simulink model "stronglyConnectedComponentsTest"  (R2021a)
settings: Solver=VariableStepDiscrete  StartTime=0.0  StopTime=10.0  RelTol=1e-3
settings Model: Creator=cyarp  LastModifiedBy=cyarp

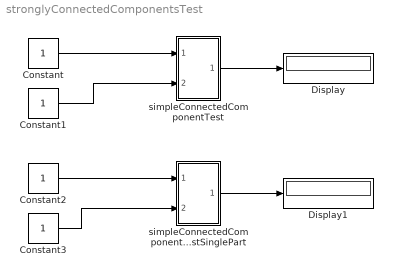
== system stronglyConnectedComponentsTest ==
  Constant{,1..3} (4 alike) : Constant  OutDataTypeStr=single
  Display : Display
  Display1 : Display
  simpleConnectedComponentTest : Subsystem
  simpleConnectedComponentTestSinglePart : Subsystem
  wires:
  Constant/1 -> simpleConnectedComponentTest/1(In1)
  Constant1/1 -> simpleConnectedComponentTest/2(In2)
  simpleConnectedComponentTest/1(Out1) -> Display/1
  Constant2/1 -> simpleConnectedComponentTestSinglePart/1(In1)
  Constant3/1 -> simpleConnectedComponentTestSinglePart/2(In2)
  simpleConnectedComponentTestSinglePart/1(Out1) -> Display1/1

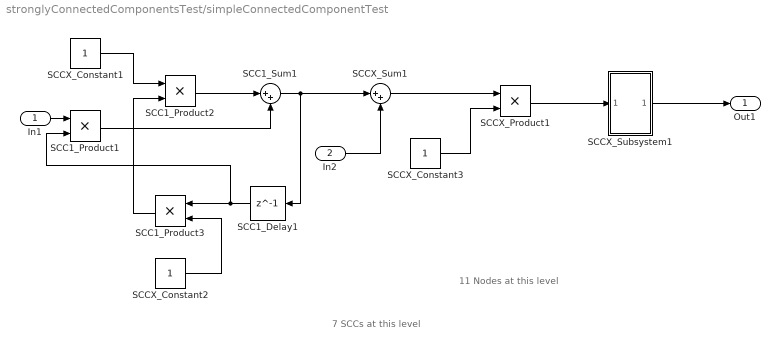
== system stronglyConnectedComponentsTest/simpleConnectedComponentTest ==
  note: 7 SCCs at this level
  note: 11 Nodes at this level
  In1 : Inport
  In2 : Inport  Port=2
  SCC1_Delay1 : Delay  DelayLength=1
  SCC1_Product1 : Product
  SCC1_Product2 : Product
  SCC1_Product3 : Product
  SCC1_Sum1 : Sum  Inputs=|++
  SCCX_Constant1 : Constant  OutDataTypeStr=single
  SCCX_Constant2 : Constant  OutDataTypeStr=single
  SCCX_Constant3 : Constant  OutDataTypeStr=single
  SCCX_Product1 : Product
  SCCX_Subsystem1 : Subsystem
  SCCX_Sum1 : Sum  Inputs=|++
  Out1 : Outport
  wires:
  SCC1_Product1/1 -> SCC1_Sum1/2
  SCC1_Delay1/1 -> SCC1_Product3/1, SCC1_Product1/2
  In2/1 -> SCCX_Sum1/2
  SCCX_Subsystem1/1(Out1) -> Out1/1
  SCC1_Sum1/1 -> SCCX_Sum1/1, SCC1_Delay1/1
  In1/1 -> SCC1_Product1/1
  SCC1_Product2/1 -> SCC1_Sum1/1
  SCCX_Sum1/1 -> SCCX_Product1/1
  SCC1_Product3/1 -> SCC1_Product2/2
  SCCX_Constant1/1 -> SCC1_Product2/1
  SCCX_Constant2/1 -> SCC1_Product3/2
  SCCX_Constant3/1 -> SCCX_Product1/2
  SCCX_Product1/1 -> SCCX_Subsystem1/1(In1)

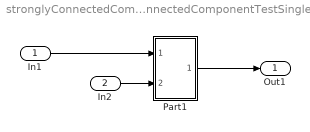
== system stronglyConnectedComponentsTest/simpleConnectedComponentTestSinglePart ==
  In1 : Inport
  In2 : Inport  Port=2
  Part1 : Subsystem
  Out1 : Outport
  wires:
  In1/1 -> Part1/1(In1)
  In2/1 -> Part1/2(In2)
  Part1/1(Out1) -> Out1/1

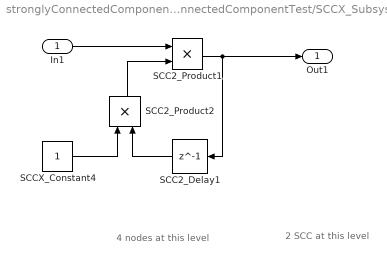
== system stronglyConnectedComponentsTest/simpleConnectedComponentTest/SCCX_Subsystem1 ==
  note: 2 SCC at this level
  note: 4 nodes at this level
  In1 : Inport
  SCC2_Delay1 : Delay  DelayLength=1
  SCC2_Product1 : Product
  SCC2_Product2 : Product
  SCCX_Constant4 : Constant  OutDataTypeStr=single
  Out1 : Outport
  wires:
  SCC2_Delay1/1 -> SCC2_Product2/2
  SCC2_Product1/1 -> Out1/1, SCC2_Delay1/1
  In1/1 -> SCC2_Product1/1
  SCC2_Product2/1 -> SCC2_Product1/2
  SCCX_Constant4/1 -> SCC2_Product2/1

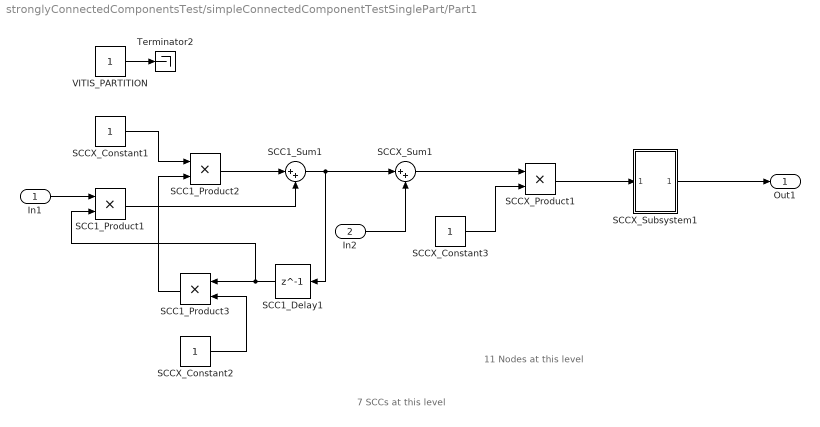
== system stronglyConnectedComponentsTest/simpleConnectedComponentTestSinglePart/Part1 ==
  note: 7 SCCs at this level
  note: 11 Nodes at this level
  In1 : Inport
  In2 : Inport  Port=2
  SCC1_Delay1 : Delay  DelayLength=1
  SCC1_Product1 : Product
  SCC1_Product2 : Product
  SCC1_Product3 : Product
  SCC1_Sum1 : Sum  Inputs=|++
  SCCX_Constant1 : Constant  OutDataTypeStr=single
  SCCX_Constant2 : Constant  OutDataTypeStr=single
  SCCX_Constant3 : Constant  OutDataTypeStr=single
  SCCX_Product1 : Product
  SCCX_Subsystem1 : Subsystem
  SCCX_Sum1 : Sum  Inputs=|++
  Terminator2 : Terminator
  VITIS_PARTITION : Constant
  Out1 : Outport
  wires:
  SCCX_Constant3/1 -> SCCX_Product1/2
  SCCX_Subsystem1/1(Out1) -> Out1/1
  SCC1_Product2/1 -> SCC1_Sum1/1
  SCC1_Delay1/1 -> SCC1_Product3/1, SCC1_Product1/2
  SCC1_Product3/1 -> SCC1_Product2/2
  SCCX_Constant2/1 -> SCC1_Product3/2
  In2/1 -> SCCX_Sum1/2
  SCC1_Sum1/1 -> SCCX_Sum1/1, SCC1_Delay1/1
  SCC1_Product1/1 -> SCC1_Sum1/2
  In1/1 -> SCC1_Product1/1
  SCCX_Constant1/1 -> SCC1_Product2/1
  SCCX_Sum1/1 -> SCCX_Product1/1
  SCCX_Product1/1 -> SCCX_Subsystem1/1(In1)
  VITIS_PARTITION/1 -> Terminator2/1

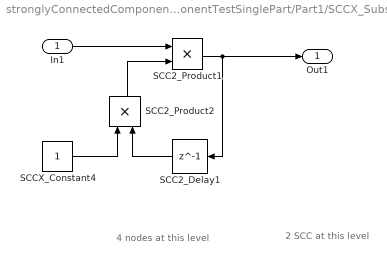
== system stronglyConnectedComponentsTest/simpleConnectedComponentTestSinglePart/Part1/SCCX_Subsystem1 ==
  note: 2 SCC at this level
  note: 4 nodes at this level
  In1 : Inport
  SCC2_Delay1 : Delay  DelayLength=1
  SCC2_Product1 : Product
  SCC2_Product2 : Product
  SCCX_Constant4 : Constant  OutDataTypeStr=single
  Out1 : Outport
  wires:
  SCC2_Delay1/1 -> SCC2_Product2/2
  SCC2_Product1/1 -> Out1/1, SCC2_Delay1/1
  In1/1 -> SCC2_Product1/1
  SCC2_Product2/1 -> SCC2_Product1/2
  SCCX_Constant4/1 -> SCC2_Product2/1
